simulink model "Push_pull"  (R2022b)
settings: Solver=VariableStepAuto  StartTime=0.0  StopTime=0.1  FixedStep=1/2e6  RelTol=1e-3
libraries: spsSeriesRLCBranchLib x6, spsCurrentMeasurementLib x3, spsMeanLib x3, spsVoltageMeasurementLib x3, spsDiodeLib x2, spsIdealSwitchLib x2, spsDCVoltageSourceLib x1, spsGroundLib x1, spsMultiWindingTransformerLib x1, spspowerguiLib x1
settings Model: Creator=smlmc  LastModifiedBy=eness
settings DebuggingCC: MaskedZcDiagnostic=none  IgnoredZcDiagnostic=none

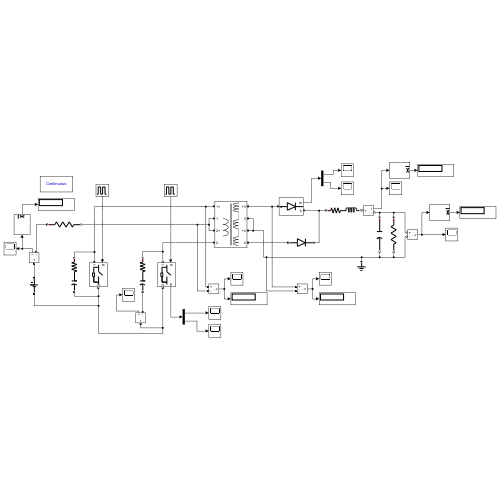
[thumbnail: Simulink's stored preview of the top-level diagram]
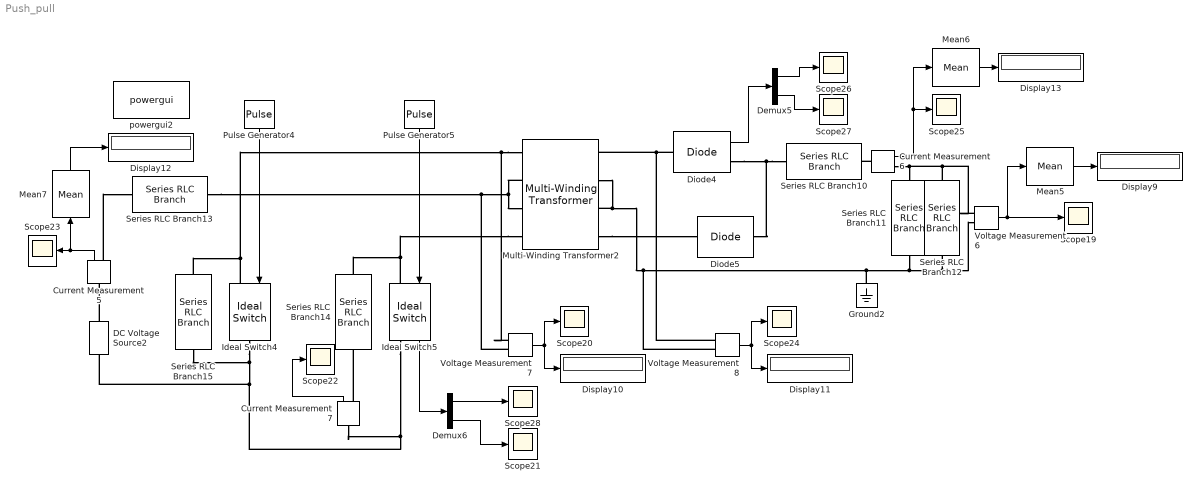
== system Push_pull ==
  Current Measurement5 : spsCurrentMeasurementLib/Current Measurement  PhasorSimulation=off  OutputType=Complex  PSBequivalent=0
  Current Measurement6 : spsCurrentMeasurementLib/Current Measurement  PhasorSimulation=off  OutputType=Complex  PSBequivalent=0
  Current Measurement7 : spsCurrentMeasurementLib/Current Measurement  PhasorSimulation=off  OutputType=Complex  PSBequivalent=0
  DC Voltage Source2 : spsDCVoltageSourceLib/DC Voltage Source  Amplitude=12  Measurements=None
  Demux5 : Demux  Outputs=2
  Demux6 : Demux  Outputs=2
  Diode4 : spsDiodeLib/Diode  Ron=0.001  Lon=0  Vf=0.1  IC=0  UseSnubber=0  Rs=inf  Cs=0  Measurements=on
  Diode5 : spsDiodeLib/Diode  Ron=0.001  Lon=0  Vf=0.1  IC=0  UseSnubber=0  Rs=inf  Cs=0  Measurements=off
  Display{9..13} (5 alike) : Display
  Ground2 : spsGroundLib/Ground  LConnTagsString=a
  Ideal Switch4 : spsIdealSwitchLib/Ideal Switch  Ron=0.0033  Lon=0  IC=0  Rs=1e5  Cs=inf  Measurements=off
  Ideal Switch5 : spsIdealSwitchLib/Ideal Switch  Ron=0.0033  Lon=0  IC=0  Rs=1e5  Cs=inf  Measurements=on
  Mean5 : spsMeanLib/Mean  Freq=60  Vinit=0  Ts=0
  Mean6 : spsMeanLib/Mean  Freq=60  Vinit=0  Ts=0
  Mean7 : spsMeanLib/Mean  Freq=60  Vinit=0  Ts=0
  Multi-Winding Transformer2 : spsMultiWindingTransformerLib/Multi-Winding Transformer  LeftWindings=2  RightWindings=2  TappedWindings=no taps  NumberOfTaps=2  SetSaturation=off  Hysteresis=off  DataFile='hysteresis.mat'  Measurements=None  UNITS=SI  NominalPower=[21.44 40e3]  NominalVoltages=[7 7 31 31]  WindingResistances=[0.0059 0.0059 0.0528 0.0528]  WindingInductances=[5.62e-8 5.62e-8 1.1e-6 1.1e-6]  Rm=27.17  Lm=93.1e-6  Saturation=[0 0;3 9.727e-11;1250 1.2321e-10]  SpecifyInitialFlux=off  InitialFlux=0  BreakLoop=off  DiscreteSolver=Trapezoidal iterative  DataType=on  TransfoNumber=1
  Pulse Generator4 : DiscretePulseGenerator  PulseType=Time based  Period=1/40e3  PulseWidth=45
  Pulse Generator5 : DiscretePulseGenerator  PulseType=Time based  Period=1/40e3  PulseWidth=45  PhaseDelay=1/80e3
  Scope{19..28} (10 alike) : Scope
  Series RLC Branch10 : spsSeriesRLCBranchLib/Series RLC Branch  LConnTagsString=__new0  RConnTagsString=__new0  BranchType=RL  Resistance=0.001  Inductance=4e-3  SetiL0=off  InitialCurrent=0  Capacitance=1e-6  Setx0=off  InitialVoltage=0  Measurements=Branch voltage and current
  Series RLC Branch11 : spsSeriesRLCBranchLib/Series RLC Branch  LConnTagsString=__new0  RConnTagsString=__new0  BranchType=C  Resistance=1  Inductance=1e-3  SetiL0=off  InitialCurrent=0  Capacitance=1.628e-8  Setx0=off  InitialVoltage=0  Measurements=None
  Series RLC Branch12 : spsSeriesRLCBranchLib/Series RLC Branch  LConnTagsString=__new0  RConnTagsString=__new0  BranchType=R  Resistance=184  Inductance=1e-3  SetiL0=off  InitialCurrent=0  Capacitance=1e-6  Setx0=off  InitialVoltage=0  Measurements=None
  Series RLC Branch13 : spsSeriesRLCBranchLib/Series RLC Branch  LConnTagsString=__new0  RConnTagsString=__new0  BranchType=R  Resistance=0.0001  Inductance=1e-3  SetiL0=off  InitialCurrent=0  Capacitance=1e-6  Setx0=off  InitialVoltage=0  Measurements=None
  Series RLC Branch14 : spsSeriesRLCBranchLib/Series RLC Branch  LConnTagsString=__new0  RConnTagsString=__new0  BranchType=RC  Resistance=4  Inductance=1e-3  SetiL0=off  InitialCurrent=0  Capacitance=47e-9  Setx0=off  InitialVoltage=0  Measurements=None
  Series RLC Branch15 : spsSeriesRLCBranchLib/Series RLC Branch  LConnTagsString=__new0  RConnTagsString=__new0  BranchType=RC  Resistance=4  Inductance=1e-3  SetiL0=off  InitialCurrent=0  Capacitance=47e-9  Setx0=off  InitialVoltage=0  Measurements=None
  Voltage Measurement6 : spsVoltageMeasurementLib/Voltage Measurement  PhasorSimulation=off  OutputType=Complex  PSBequivalent=0
  Voltage Measurement7 : spsVoltageMeasurementLib/Voltage Measurement  PhasorSimulation=off  OutputType=Complex  PSBequivalent=0
  Voltage Measurement8 : spsVoltageMeasurementLib/Voltage Measurement  PhasorSimulation=off  OutputType=Complex  PSBequivalent=0
  powergui2 : spspowerguiLib/powergui  Priority=1  SimulationMode=Continuous  SampleTime=50e-6  frequency=60  Iterations=50  frequencyindice=0  Pbase=100e6  ErrMax=1e-4  UnitsV=kV  UnitsW=MW  buscounter=0  FunctionMessages=off  echomessages=off  EnableUseOfTLC=off  CurrentSourceSwitches=off  DisableSnubberDevices=off  DisableRonSwitches=off  DisableVfSwitches=off  DisplayEquations=off  AutomaticDiscreteSolvers=off  SolverType=Tustin/Backward Euler (TBE)  Interpol=off  ExternalGateDelay=off  methode=off  Ts=100  x0status=blocks  SPID=on  SwTol=0  HookPort=off  NonlinearTolerance=1e-4  nMaxIteration=100  ContinueOnMaxIteration=off  RestoreLinks=warning  ResistiveCurrentMeasurement=off  Frange=[0:2:500]  Ylog=off  Xlog=on  ShowGrid=off  save=off  variable=ZData  structure=0  ZoomFFT=off  StartTime=0.0  cycles=1  DisplayStyle=1  fundamental=60  FreqAxis=off  MaxFrequency=1000  frequencyindicesteady=1  RmsSteady=1  display=off
  wires:
  Demux6/1 -> Scope28/1
  Voltage Measurement6/1 -> Mean5/1, Scope19/1
  Current Measurement7/1 -> Scope22/1
  Pulse Generator4/1 -> Ideal Switch4/1
  Current Measurement6/1 -> Mean6/1, Scope25/1
  Mean6/1 -> Display13/1
  Pulse Generator5/1 -> Ideal Switch5/1
  Current Measurement5/1 -> Mean7/1, Scope23/1
  Mean7/1 -> Display12/1
  Diode4/1 -> Demux5/1
  Voltage Measurement8/1 -> Scope24/1, Display11/1
  Demux6/2 -> Scope21/1
  Demux5/1 -> Scope26/1
  Voltage Measurement7/1 -> Scope20/1, Display10/1
  Mean5/1 -> Display9/1
  Demux5/2 -> Scope27/1
  Ideal Switch5/1 -> Demux6/1
  connections:
  Ground2/LConn1 -- Voltage Measurement6/LConn2 -- Series RLC Branch12/RConn1 -- Series RLC Branch11/RConn1 -- Multi-Winding Transformer2/RConn2 -- Multi-Winding Transformer2/RConn3 -- Voltage Measurement8/LConn2
  Multi-Winding Transformer2/LConn4 -- Ideal Switch5/LConn1 -- Series RLC Branch14/LConn1
  Series RLC Branch13/RConn1 -- Voltage Measurement7/LConn2 -- Multi-Winding Transformer2/LConn2 -- Multi-Winding Transformer2/LConn3
  Series RLC Branch10/LConn1 -- Diode4/RConn1 -- Diode5/RConn1
  Voltage Measurement8/LConn1 -- Multi-Winding Transformer2/RConn1 -- Diode4/LConn1
  DC Voltage Source2/LConn1 -- Current Measurement7/LConn1 -- Ideal Switch5/RConn1 -- Ideal Switch4/RConn1 -- Series RLC Branch15/RConn1
  Multi-Winding Transformer2/LConn1 -- Voltage Measurement7/LConn1 -- Series RLC Branch15/LConn1 -- Ideal Switch4/LConn1
  Series RLC Branch12/LConn1 -- Voltage Measurement6/LConn1 -- Series RLC Branch11/LConn1 -- Current Measurement6/RConn1
  Current Measurement7/RConn1 -- Series RLC Branch14/RConn1
  Multi-Winding Transformer2/RConn4 -- Diode5/LConn1
  Current Measurement6/LConn1 -- Series RLC Branch10/RConn1
  Current Measurement5/RConn1 -- Series RLC Branch13/LConn1
  DC Voltage Source2/RConn1 -- Current Measurement5/LConn1
